simulink model "CubeX_Fast_MPC_2D"  (R2016b)
settings: Solver=FixedStepDiscrete  StartTime=0.0  StopTime=inf  FixedStep=Ts.base  RelTol=1e-3
PreLoadFcn:
  | waijung.modelPreload; % Required for working with Waijung Blockset. Do not remove.
InitFcn:
  | cubeparameters
undefined symbols (not defined in the file or in its folder): CPHA_1Edge, CPOL_Low, deg_, Duplex, FirstBit_MSB, Full, g, imu, Link, LQFP100, ST, STM32F407VG, STM32F4DISCOVERY, Ts
libraries: simulink x47, stm32f4_i2c_lib x12, stm32f4_io_lib x5, stm32f4_spi_lib x4, cube_lib x3, BC_USB x2, stm32f4_adc_lib x1, stm32f4_device_config_lib x1
(part 2 of 3)

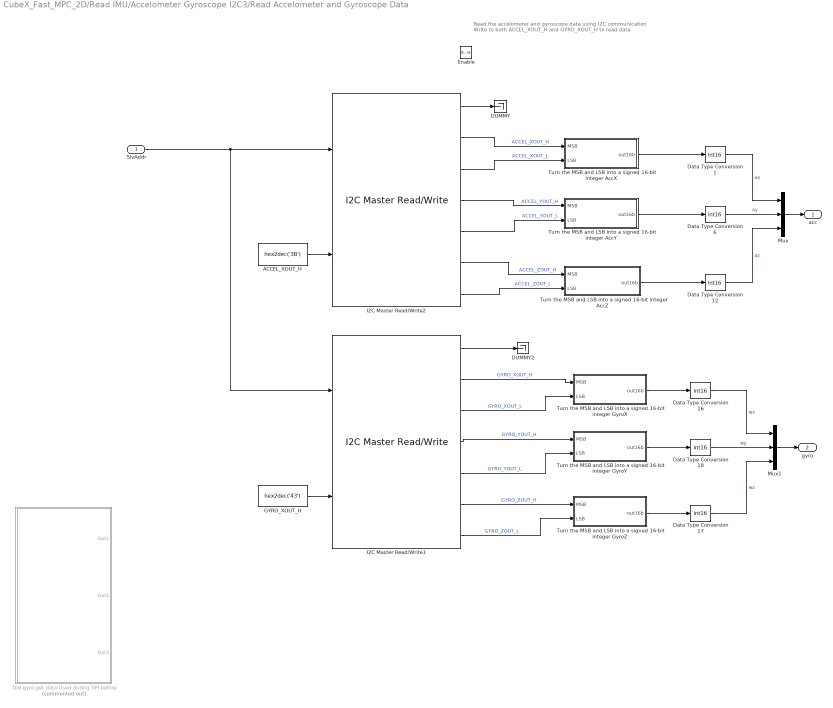
== system CubeX_Fast_MPC_2D/Read IMU/Accelometer Gyroscope I2C3/Read Accelometer and Gyroscope Data ==
  note: Read the accelometer and gyroscope data using I2C communication
      | Write to both ACCEL_XOUT_H and GYRO_XOUT_H to read data
  SlvAddr : Inport
  Enable : EnablePort
  ACCEL_XOUT_H : Constant  Value=hex2dec('3B')  OutDataTypeStr=uint8  SampleTime=-1
  DUMMY : Terminator
  DUMMY2 : Terminator
  Data Type Conversion{1,6,12,16..18} (6 alike) : DataTypeConversion  OutDataTypeStr=int16
  GYRO_XOUT_H : Constant  Value=hex2dec('43')  OutDataTypeStr=uint8  SampleTime=-1
  I2C Master Read/Write1 : stm32f4_i2c_lib/I2C Master Read//Write  configuration=Transaction  module=3  lastmodule=3  transfer=Blocking  dutycycle=TLow/THigh = 2  clkspeed=400  timeout=25  writecount=1  readcount=6  sdapin=C9  sclpin=A8  waitwritetime=0  forcestop=off  inputtypearray=[2 3 3]  outputtypearray=[7 3 3 3 3 3 3 3]  confstr="[\"C\",\"9\",\"A\",\"8\",\"1\",\"3\",\"4\",\"2\",\"I2C_DutyCycle_2\",\"0\",\"off\"]"  sampletime=Ts.IMU  sampletimestr=0.008  blockid=ReadIMUAccelometerGyroscopeI2C3ReadAccelometerandGyroscopeDataI2CMasterReadWrite1
  I2C Master Read/Write2 : stm32f4_i2c_lib/I2C Master Read//Write  configuration=Transaction  module=3  lastmodule=3  transfer=Blocking  dutycycle=TLow/THigh = 2  clkspeed=400  timeout=25  writecount=1  readcount=6  sdapin=C9  sclpin=A8  waitwritetime=0  forcestop=off  inputtypearray=[2 3 3]  outputtypearray=[7 3 3 3 3 3 3 3]  confstr="[\"C\",\"9\",\"A\",\"8\",\"1\",\"3\",\"4\",\"2\",\"I2C_DutyCycle_2\",\"0\",\"off\"]"  sampletime=Ts.IMU  sampletimestr=0.008  blockid=ReadIMUAccelometerGyroscopeI2C3ReadAccelometerandGyroscopeDataI2CMasterReadWrite2
  Mux : Mux  Inputs=3
  Mux1 : Mux  Inputs=3
  Old gyro get data Used during SPI before : Subsystem  Commented=on
  Turn the MSB and LSB into a signed 16-bit integer AccX : Subsystem
  Turn the MSB and LSB into a signed 16-bit integer AccY : Subsystem
  Turn the MSB and LSB into a signed 16-bit integer AccZ : Subsystem
  Turn the MSB and LSB into a signed 16-bit integer GyroX : Subsystem
  Turn the MSB and LSB into a signed 16-bit integer GyroY : Subsystem
  Turn the MSB and LSB into a signed 16-bit integer GyroZ : Subsystem
  acc : Outport
  gyro : Outport  Port=2
  wires:
  I2C Master Read/Write2/1 -> DUMMY/1
  Mux/1 -> acc/1
  Turn the MSB and LSB into a signed 16-bit integer AccX/1(out16b) -> Data Type Conversion1/1
  Turn the MSB and LSB into a signed 16-bit integer AccY/1(out16b) -> Data Type Conversion6/1
  Turn the MSB and LSB into a signed 16-bit integer AccZ/1(out16b) -> Data Type Conversion12/1
  Data Type Conversion1/1 -> Mux/1  "ax"
  Data Type Conversion6/1 -> Mux/2  "ay"
  Data Type Conversion12/1 -> Mux/3  "az"
  I2C Master Read/Write1/1 -> DUMMY2/1
  Mux1/1 -> gyro/1
  Turn the MSB and LSB into a signed 16-bit integer GyroX/1(out16b) -> Data Type Conversion16/1
  Turn the MSB and LSB into a signed 16-bit integer GyroY/1(out16b) -> Data Type Conversion18/1
  Turn the MSB and LSB into a signed 16-bit integer GyroZ/1(out16b) -> Data Type Conversion17/1
  Data Type Conversion16/1 -> Mux1/1  "wx"
  Data Type Conversion18/1 -> Mux1/2  "wy"
  Data Type Conversion17/1 -> Mux1/3  "wz"
  GYRO_XOUT_H/1 -> I2C Master Read/Write1/2
  ACCEL_XOUT_H/1 -> I2C Master Read/Write2/2
  SlvAddr/1 -> I2C Master Read/Write1/1, I2C Master Read/Write2/1
  I2C Master Read/Write2/2 -> Turn the MSB and LSB into a signed 16-bit integer AccX/1(MSB)  "ACCEL_XOUT_H"
  I2C Master Read/Write2/3 -> Turn the MSB and LSB into a signed 16-bit integer AccX/2(LSB)  "ACCEL_XOUT_L"
  I2C Master Read/Write2/5 -> Turn the MSB and LSB into a signed 16-bit integer AccY/2(LSB)  "ACCEL_YOUT_L"
  I2C Master Read/Write2/4 -> Turn the MSB and LSB into a signed 16-bit integer AccY/1(MSB)  "ACCEL_YOUT_H"
  I2C Master Read/Write2/6 -> Turn the MSB and LSB into a signed 16-bit integer AccZ/1(MSB)  "ACCEL_ZOUT_H"
  I2C Master Read/Write2/7 -> Turn the MSB and LSB into a signed 16-bit integer AccZ/2(LSB)  "ACCEL_ZOUT_L"
  I2C Master Read/Write1/2 -> Turn the MSB and LSB into a signed 16-bit integer GyroX/1(MSB)  "GYRO_XOUT_H"
  I2C Master Read/Write1/3 -> Turn the MSB and LSB into a signed 16-bit integer GyroX/2(LSB)  "GYRO_XOUT_L"
  I2C Master Read/Write1/4 -> Turn the MSB and LSB into a signed 16-bit integer GyroY/1(MSB)  "GYRO_YOUT_H"
  I2C Master Read/Write1/5 -> Turn the MSB and LSB into a signed 16-bit integer GyroY/2(LSB)  "GYRO_YOUT_L"
  I2C Master Read/Write1/6 -> Turn the MSB and LSB into a signed 16-bit integer GyroZ/1(MSB)  "GYRO_ZOUT_H"
  I2C Master Read/Write1/7 -> Turn the MSB and LSB into a signed 16-bit integer GyroZ/2(LSB)  "GYRO_ZOUT_L"

== system CubeX_Fast_MPC_2D/Read IMU/Magnetometer I2C1/AK8963 Init  ==
  note: See if the magnetometer is on, if not
      | set the mode to  Continuous measurement mode 2 and the output to 16 bits
      | in Write Configuration
  SlvAddr : Inport
  AK8963_CNTL : Constant  Value=hex2dec('0A')  OutDataTypeStr=uint8  SampleTime=-1
  Bitwise Operator : simulink/Logic and Bit Operations/Bitwise Operator  logicop=AND  UseBitMask=on  BitMask=bin2dec('00010110')  BitMaskRealWorld=Stored Integer
  Compare To Zero : simulink/Logic and Bit Operations/Compare To Zero  relop===  OutDataTypeStr=boolean
  I2C Master Read/Write : stm32f4_i2c_lib/I2C Master Read//Write  configuration=Transaction  module=1  lastmodule=3  transfer=Blocking  dutycycle=TLow/THigh = 2  clkspeed=400  timeout=25  writecount=1  readcount=1  sdapin=C9  sclpin=A8  waitwritetime=0  forcestop=off  inputtypearray=[2 3 3]  outputtypearray=[2 3 3]  confstr="[\"C\",\"9\",\"A\",\"8\",\"1\",\"1\",\"6\",\"0\",\"I2C_DutyCycle_2\",\"0\",\"off\"]"  sampletime=-1  sampletimestr=0.002  blockid=ReadIMUMagnetometerI2CAK8963InitI2CMasterReadWrite
  Logical Operator : Logic  AllPortsSameDT=off  OutDataTypeStr=boolean
  Logical Operator1 : Logic  AllPortsSameDT=off  OutDataTypeStr=boolean
  Logical Operator2 : Logic  Operator=NOT  AllPortsSameDT=off  OutDataTypeStr=boolean
  Write Configuration : Subsystem
  READY : Outport
  wires:
  SlvAddr/1 -> Write Configuration/1(SlvAddr), I2C Master Read/Write/1
  AK8963_CNTL/1 -> Write Configuration/2(RegAddr), I2C Master Read/Write/2
  I2C Master Read/Write/1 -> Compare To Zero/1
  Logical Operator/1 -> READY/1
  Bitwise Operator/1 -> Logical Operator2/1, Logical Operator/2
  Compare To Zero/1 -> Logical Operator/1, Logical Operator1/1
  I2C Master Read/Write/2 -> Bitwise Operator/1
  Logical Operator2/1 -> Logical Operator1/2
  Logical Operator1/1 -> Write Configuration/Enable

== system CubeX_Fast_MPC_2D/Read IMU/Magnetometer I2C1/Magnetometer Data Ready  ==
  note: Check if magnetometer data is ready
  SlvAddr : Inport
  Enable : EnablePort
  AK8963_ST1 : Constant  Value=hex2dec('02')  OutDataTypeStr=uint8  SampleTime=-1
  Bitwise Operator : simulink/Logic and Bit Operations/Bitwise Operator  logicop=AND  UseBitMask=on  BitMask=bin2dec('00000001')  BitMaskRealWorld=Stored Integer
  Compare To Zero : simulink/Logic and Bit Operations/Compare To Zero  relop===  OutDataTypeStr=boolean
  I2C Master Read/Write : stm32f4_i2c_lib/I2C Master Read//Write  configuration=Transaction  module=1  lastmodule=3  transfer=Blocking  dutycycle=TLow/THigh = 2  clkspeed=400  timeout=25  writecount=1  readcount=1  sdapin=C9  sclpin=A8  waitwritetime=0  forcestop=off  inputtypearray=[2 3 3]  outputtypearray=[2 3 3]  confstr="[\"C\",\"9\",\"A\",\"8\",\"1\",\"1\",\"6\",\"0\",\"I2C_DutyCycle_2\",\"0\",\"off\"]"  sampletime=-1  sampletimestr=0.002  blockid=ReadIMUMagnetometerI2CMagnetometerDataReadyI2CMasterReadWrite
  Logical Operator : Logic  AllPortsSameDT=off  OutDataTypeStr=boolean
  READY : Outport
  wires:
  SlvAddr/1 -> I2C Master Read/Write/1
  AK8963_ST1/1 -> I2C Master Read/Write/2
  I2C Master Read/Write/2 -> Bitwise Operator/1
  I2C Master Read/Write/1 -> Compare To Zero/1
  Compare To Zero/1 -> Logical Operator/1
  Bitwise Operator/1 -> Logical Operator/2
  Logical Operator/1 -> READY/1

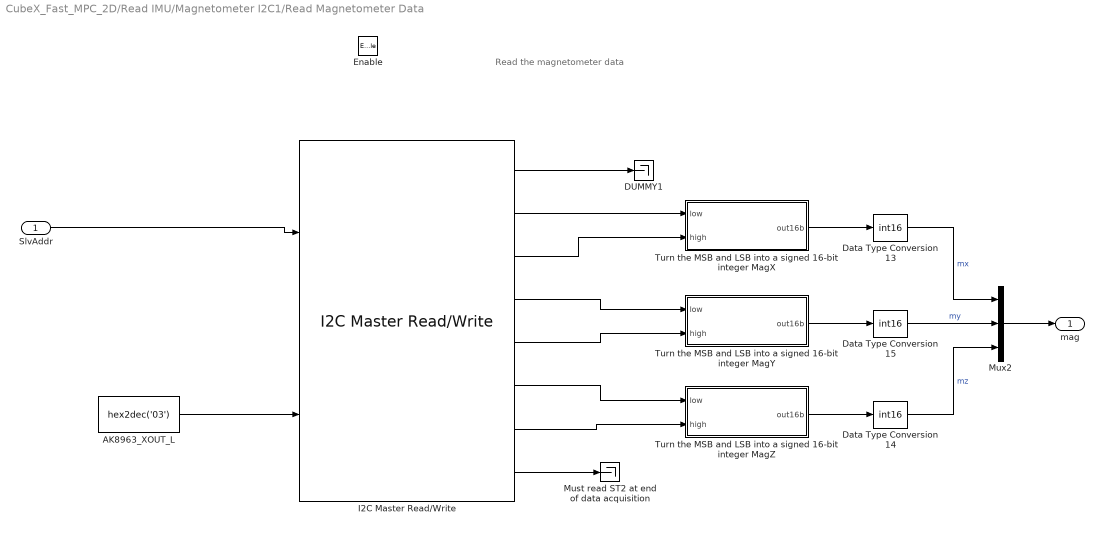
== system CubeX_Fast_MPC_2D/Read IMU/Magnetometer I2C1/Read Magnetometer Data ==
  note: Read the magnetometer data
  "SlvAddr " : Inport
  Enable : EnablePort
  AK8963_XOUT_L : Constant  Value=hex2dec('03')  OutDataTypeStr=uint8  SampleTime=-1
  DUMMY1 : Terminator
  Data Type Conversion13 : DataTypeConversion  OutDataTypeStr=int16
  Data Type Conversion14 : DataTypeConversion  OutDataTypeStr=int16
  Data Type Conversion15 : DataTypeConversion  OutDataTypeStr=int16
  I2C Master Read/Write : stm32f4_i2c_lib/I2C Master Read//Write  configuration=Transaction  module=1  lastmodule=3  transfer=Blocking  dutycycle=TLow/THigh = 2  clkspeed=400  timeout=25  writecount=1  readcount=7  sdapin=C9  sclpin=A8  waitwritetime=0  forcestop=off  inputtypearray=[2 3 3]  outputtypearray=[8 3 3 3 3 3 3 3 3]  confstr="[\"C\",\"9\",\"A\",\"8\",\"1\",\"1\",\"6\",\"0\",\"I2C_DutyCycle_2\",\"0\",\"off\"]"  sampletime=-1  sampletimestr=0.002  blockid=ReadIMUMagnetometerI2CReadMagnetometerDataI2CMasterReadWrite
  "Must read ST2 at end of data acquisition  " : Terminator
  Mux2 : Mux  Inputs=3
  Turn the MSB and LSB into a signed 16-bit integer MagX : Subsystem
  Turn the MSB and LSB into a signed 16-bit integer MagY : Subsystem
  Turn the MSB and LSB into a signed 16-bit integer MagZ : Subsystem
  mag : Outport
  wires:
  Turn the MSB and LSB into a signed 16-bit integer MagX/1(out16b) -> Data Type Conversion13/1
  Turn the MSB and LSB into a signed 16-bit integer MagY/1(out16b) -> Data Type Conversion15/1
  Turn the MSB and LSB into a signed 16-bit integer MagZ/1(out16b) -> Data Type Conversion14/1
  Data Type Conversion13/1 -> Mux2/1  "mx"
  Data Type Conversion15/1 -> Mux2/2  "my"
  Data Type Conversion14/1 -> Mux2/3  "mz"
  AK8963_XOUT_L/1 -> I2C Master Read/Write/2
  I2C Master Read/Write/1 -> DUMMY1/1
  "SlvAddr "/1 -> I2C Master Read/Write/1
  Mux2/1 -> mag/1
  I2C Master Read/Write/8 -> "Must read ST2 at end of data acquisition  "/1
  I2C Master Read/Write/3 -> Turn the MSB and LSB into a signed 16-bit integer MagX/2(high)
  I2C Master Read/Write/2 -> Turn the MSB and LSB into a signed 16-bit integer MagX/1(low)
  I2C Master Read/Write/4 -> Turn the MSB and LSB into a signed 16-bit integer MagY/1(low)
  I2C Master Read/Write/5 -> Turn the MSB and LSB into a signed 16-bit integer MagY/2(high)
  I2C Master Read/Write/6 -> Turn the MSB and LSB into a signed 16-bit integer MagZ/1(low)
  I2C Master Read/Write/7 -> Turn the MSB and LSB into a signed 16-bit integer MagZ/2(high)

== system CubeX_Fast_MPC_2D/Read IMU/SPI3/Turn the MSB and LSB into a signed 16-bit integer AccX ==
  MSB : Inport
  LSB : Inport  Port=2
  Bitwise Operator2 : simulink/Logic and Bit Operations/Bitwise Operator  logicop=OR  UseBitMask=off  NumInputPorts=2  BitMask=bin2dec('11011001')  BitMaskRealWorld=Stored Integer
  Data Type Conversion6 : DataTypeConversion  OutDataTypeStr=uint16
  Data Type Conversion7 : DataTypeConversion  OutDataTypeStr=uint16
  Shift Arithmetic2 : ArithShift  BitShiftNumber=-8
  out16b : Outport
  wires:
  LSB/1 -> Data Type Conversion6/1
  Bitwise Operator2/1 -> out16b/1
  MSB/1 -> Data Type Conversion7/1
  Data Type Conversion7/1 -> Shift Arithmetic2/1
  Data Type Conversion6/1 -> Bitwise Operator2/2
  Shift Arithmetic2/1 -> Bitwise Operator2/1

== system CubeX_Fast_MPC_2D/Read IMU/SPI3/Turn the MSB and LSB into a signed 16-bit integer AccY ==
  MSB : Inport
  LSB : Inport  Port=2
  Bitwise Operator2 : simulink/Logic and Bit Operations/Bitwise Operator  logicop=OR  UseBitMask=off  NumInputPorts=2  BitMask=bin2dec('11011001')  BitMaskRealWorld=Stored Integer
  Data Type Conversion6 : DataTypeConversion  OutDataTypeStr=int16
  Data Type Conversion7 : DataTypeConversion  OutDataTypeStr=int16
  Shift Arithmetic2 : ArithShift  BitShiftNumber=-8
  out16b : Outport
  wires:
  LSB/1 -> Data Type Conversion6/1
  Bitwise Operator2/1 -> out16b/1
  MSB/1 -> Data Type Conversion7/1
  Data Type Conversion7/1 -> Shift Arithmetic2/1
  Data Type Conversion6/1 -> Bitwise Operator2/2
  Shift Arithmetic2/1 -> Bitwise Operator2/1

== system CubeX_Fast_MPC_2D/Read IMU/SPI3/Turn the MSB and LSB into a signed 16-bit integer AccZ ==
  MSB : Inport
  LSB : Inport  Port=2
  Bitwise Operator2 : simulink/Logic and Bit Operations/Bitwise Operator  logicop=OR  UseBitMask=off  NumInputPorts=2  BitMask=bin2dec('11011001')  BitMaskRealWorld=Stored Integer
  Data Type Conversion6 : DataTypeConversion  OutDataTypeStr=int16
  Data Type Conversion7 : DataTypeConversion  OutDataTypeStr=int16
  Shift Arithmetic2 : ArithShift  BitShiftNumber=-8
  out16b : Outport
  wires:
  LSB/1 -> Data Type Conversion6/1
  Bitwise Operator2/1 -> out16b/1
  MSB/1 -> Data Type Conversion7/1
  Data Type Conversion7/1 -> Shift Arithmetic2/1
  Data Type Conversion6/1 -> Bitwise Operator2/2
  Shift Arithmetic2/1 -> Bitwise Operator2/1

== system CubeX_Fast_MPC_2D/Read IMU/SPI3/Turn the MSB and LSB into a signed 16-bit integer GyroX ==
  MSB : Inport
  LSB : Inport  Port=2
  Bitwise Operator2 : simulink/Logic and Bit Operations/Bitwise Operator  logicop=OR  UseBitMask=off  NumInputPorts=2  BitMask=bin2dec('11011001')  BitMaskRealWorld=Stored Integer
  Data Type Conversion1 : DataTypeConversion  OutDataTypeStr=int16
  Data Type Conversion7 : DataTypeConversion  OutDataTypeStr=int16
  Shift Arithmetic2 : ArithShift  BitShiftNumber=-8
  out16b : Outport
  wires:
  MSB/1 -> Data Type Conversion7/1
  Data Type Conversion7/1 -> Shift Arithmetic2/1
  Shift Arithmetic2/1 -> Bitwise Operator2/1
  LSB/1 -> Data Type Conversion1/1
  Data Type Conversion1/1 -> Bitwise Operator2/2
  Bitwise Operator2/1 -> out16b/1

== system CubeX_Fast_MPC_2D/Read IMU/SPI3/Turn the MSB and LSB into a signed 16-bit integer GyroY ==
  MSB : Inport
  LSB : Inport  Port=2
  Bitwise Operator2 : simulink/Logic and Bit Operations/Bitwise Operator  logicop=OR  UseBitMask=off  NumInputPorts=2  BitMask=bin2dec('11011001')  BitMaskRealWorld=Stored Integer
  Data Type Conversion6 : DataTypeConversion  OutDataTypeStr=uint16
  Data Type Conversion7 : DataTypeConversion  OutDataTypeStr=uint16
  Shift Arithmetic2 : ArithShift  BitShiftNumber=-8
  out16b : Outport
  wires:
  LSB/1 -> Data Type Conversion6/1
  Bitwise Operator2/1 -> out16b/1
  MSB/1 -> Data Type Conversion7/1
  Data Type Conversion7/1 -> Shift Arithmetic2/1
  Data Type Conversion6/1 -> Bitwise Operator2/2
  Shift Arithmetic2/1 -> Bitwise Operator2/1

== system CubeX_Fast_MPC_2D/Read IMU/SPI3/Turn the MSB and LSB into a signed 16-bit integer GyroZ ==
  MSB : Inport
  LSB : Inport  Port=2
  Bitwise Operator2 : simulink/Logic and Bit Operations/Bitwise Operator  logicop=OR  UseBitMask=off  NumInputPorts=2  BitMask=bin2dec('11011001')  BitMaskRealWorld=Stored Integer
  Data Type Conversion6 : DataTypeConversion  OutDataTypeStr=uint16
  Data Type Conversion7 : DataTypeConversion  OutDataTypeStr=uint16
  Shift Arithmetic2 : ArithShift  BitShiftNumber=-8
  out16b : Outport
  wires:
  LSB/1 -> Data Type Conversion6/1
  Bitwise Operator2/1 -> out16b/1
  MSB/1 -> Data Type Conversion7/1
  Data Type Conversion7/1 -> Shift Arithmetic2/1
  Data Type Conversion6/1 -> Bitwise Operator2/2
  Shift Arithmetic2/1 -> Bitwise Operator2/1

== system CubeX_Fast_MPC_2D/Read IMU/Subsystem/Subsystem ==
  Enable : EnablePort
  SPI Master Read/Write1 : stm32f4_spi_lib/SPI Master Read//Write  configuration=Transaction  module=3  mode=Read/ Write  lastmodule=1  direction=Full-Duplex  dataformat=8bit/ FirstBit_MSB  prescaler=4  cpolcpha=CPOL_Low/ CPHA_1Edge  datacount=2  nssmode=Custom  nsspin=Not used  softnssport=E  softnsspin=0  sckpin=A5  misopin=A6  mosipin=A7  inputtypearray=[2 3 3]  outputtypearray=[3 7 3 3]  confstr="[\"SPI_Direction_2Lines_FullDuplex\",\"8b\",\"MSB\",\"Low\",\"1Edge\",\"4\",\"Soft\",\"0\",\"x\",\"x\",\"0\",\"x\",\"x\",\"1\",\"A\",\"5\",\"1\",\"A\",\"6\",\"1\",\"A\",\"7\",\"1\",\"0\",\"0\",\"0\",\"0\",\"0\",\"0\",\"0\",\"0\",\"PP\",\"0\",\"UP\"]"  sampletime=0.002  sampletimestr=0.002  blockid=ReadIMUSubsystemSubsystemSPIMasterReadWrite1
  Terminator : Terminator
  Terminator1 : Terminator
  Terminator2 : Terminator
  USER_CTRL : Constant  Value=hex2dec('6A')  OutDataTypeStr=uint8  SampleTime=-1
  USER_CTRL1 : Constant  Value=hex2dec('10')  OutDataTypeStr=uint8  SampleTime=-1
  wires:
  SPI Master Read/Write1/3 -> Terminator/1
  SPI Master Read/Write1/2 -> Terminator1/1
  SPI Master Read/Write1/1 -> Terminator2/1
  USER_CTRL/1 -> SPI Master Read/Write1/1
  USER_CTRL1/1 -> SPI Master Read/Write1/2

== system CubeX_Fast_MPC_2D/Read IMU/Accelometer Gyroscope I2C1/MPU9250 Init/Write Configuration ==
  note: Enable BYPSS_EN in INT_PIN_CFG register to be able to read magnetometer trough I2C
  SlvAddr : Inport
  Enable : EnablePort
  BYPASS_EN : Constant  Value=hex2dec('02')  OutDataTypeStr=uint8  SampleTime=-1
  I2C Master Read/Write1 : stm32f4_i2c_lib/I2C Master Read//Write  configuration=Transaction  module=1  lastmodule=3  transfer=Blocking  dutycycle=TLow/THigh = 2  clkspeed=400  timeout=25  writecount=2  readcount=0  sdapin=C9  sclpin=A8  waitwritetime=0  forcestop=off  inputtypearray=[3 3 3 3]  outputtypearray=[1 3]  confstr="[\"C\",\"9\",\"A\",\"8\",\"1\",\"1\",\"6\",\"0\",\"I2C_DutyCycle_2\",\"0\",\"off\"]"  sampletime=-1  sampletimestr=0.008  blockid=ReadIMUAccelometerGyroscopeI2C1MPU9250InitWriteConfigurationI2CMasterReadWrite1
  INT_PIN_CFG1 : Constant  Value=hex2dec('37')  OutDataTypeStr=uint8  SampleTime=-1
  Terminator : Terminator
  wires:
  I2C Master Read/Write1/1 -> Terminator/1
  BYPASS_EN/1 -> I2C Master Read/Write1/3
  INT_PIN_CFG1/1 -> I2C Master Read/Write1/2
  SlvAddr/1 -> I2C Master Read/Write1/1

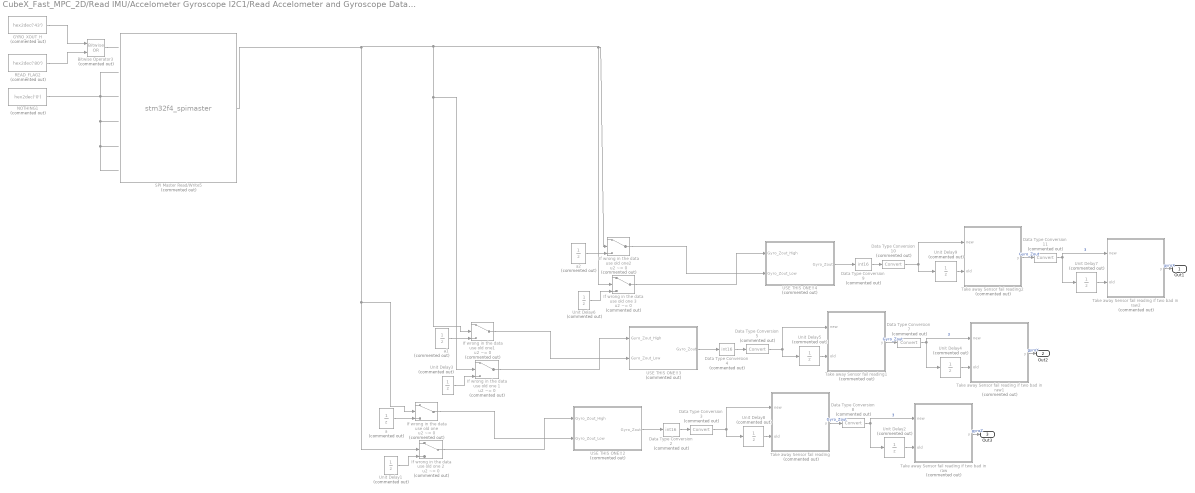
== system CubeX_Fast_MPC_2D/Read IMU/Accelometer Gyroscope I2C1/Read Accelometer and Gyroscope Data/Old gyro get data Used during SPI before ==
  " a" : UnitDelay  Commented=on  SampleTime=-1
  " a1" : UnitDelay  Commented=on  SampleTime=-1
  " a2" : UnitDelay  Commented=on  SampleTime=-1
  Bitwise Operator3 : simulink/Logic and Bit Operations/Bitwise Operator  Commented=on  logicop=OR  UseBitMask=off  NumInputPorts=2  BitMask=bin2dec('11011001')  BitMaskRealWorld=Stored Integer
  Data Type Conversion{3,5,7..8,10..11} (6 alike) : DataTypeConversion  Commented=on
  Data Type Conversion2 : DataTypeConversion  Commented=on  OutDataTypeStr=int16
  Data Type Conversion4 : DataTypeConversion  Commented=on  OutDataTypeStr=int16
  Data Type Conversion9 : DataTypeConversion  Commented=on  OutDataTypeStr=int16
  GYRO_XOUT_H : Constant  Commented=on  Value=hex2dec('43')  OutDataTypeStr=uint8
  If wrong in the data use old one : Switch  Commented=on  Criteria=u2 ~= 0
  If wrong in the data use old one 1 : Switch  Commented=on  Criteria=u2 ~= 0
  If wrong in the data use old one 2 : Switch  Commented=on  Criteria=u2 ~= 0
  If wrong in the data use old one 3 : Switch  Commented=on  Criteria=u2 ~= 0
  If wrong in the data use old one1 : Switch  Commented=on  Criteria=u2 ~= 0
  If wrong in the data use old one2 : Switch  Commented=on  Criteria=u2 ~= 0
  NOTHING1 : Constant  Commented=on  Value=hex2dec('0')  OutDataTypeStr=uint8
  READ_FLAG2 : Constant  Commented=on  Value=hex2dec('80')  OutDataTypeStr=uint8
  SPI Master Read/Write5 : S-Function  Commented=on  FunctionName=stm32f4_spimaster  Parameters=mode,configuration,module,datacount,inputtypearray,outputtypearray,confstr,sampletime,sampletimestr,blockid  SFunctionDeploymentMode=off  EnableBusSupport=off  mask(stm32f4_spimaster){configuration=Transaction, module=3, mode=Read/ Write, lastmodule=1, direction=Full-Duplex, dataformat=8bit/ FirstBit_MSB, prescaler=4, cpolcpha=CPOL_Low/ CPHA_1Edge, datacount='Could not find SPI Master Setup block for module 3', nssmode=Custom, nsspin=Not used, softnssport=E, softnsspin=0, sckpin=A5, misopin=A6, mosipin=A7, inputtypearray=[0], outputtypearray=[1 7], confstr=["SPI_Direction_2Lines_FullDuplex","8b","MSB","Low","1Edge","4","Soft","0","x","x","0","x","x","1","A","5","1","A","6","1","A","7","1","0","0","0","0","0","0","0","0","PP","0","UP"], sampletime=-1, sampletimestr=-1, blockid=AccelometerGyroscopeI2CReadAccelometerandGyroscopeDataOldgyrogetdataUsedduringSPIbeforeSPIMasterReadWrite5}
      mask prompts: module "SPI Module:"; lastmodule "Last module:"; dataformat "Data format:"; prescaler "Buad rate prescaler: Pclk/"; cpolcpha "Clock polarity (CPOL)/ Clock phase (CPHA):"; datacount "Data Read/Write count:"; nssmode "Slave/chip select (nSS, nCS) mode"; nsspin "Slave/chip select (nSS, nCS) pin"; softnssport "Slave/chip select port (nSS, nCS)"; softnsspin "Slave/chip select pin (nSS, nCS)"; sckpin "SCLK pin:"; misopin "MISO pin:"; mosipin "MOSI pin:"; inputtypearray "Input type array"; outputtypearray "Output type array"; confstr "Configuration string"; sampletime "Sample time (sec)"; sampletimestr "Compiled sample time (sec) in string"
      mask help:
      | Status:
      |  0 - Success.
      |  Otherwise - Fail.
      mask init:
      | stm32f4_spimaster_callback('init');
      mask Help: web(fullfile(waijungdocroot,'stm32f4_spimaster_readwrite.htm'), '-browser')
      mask TypeOptions configuration: Setup | Transaction
      mask Callback configuration: stm32f4_spimaster_callback('configuration');
      mask TypeOptions module: 1 | 2 | 3
      mask Callback module: stm32f4_spimaster_callback('module');
      mask TypeOptions mode: Read/ Write | Read | Write
      mask Callback mode: stm32f4_spimaster_callback('mode');
      mask TypeOptions direction: Full-Duplex | Half-Duplex_Tx | Half-Duplex_Rx
      mask Callback direction: stm32f4_spimaster_callback('direction');
      mask TypeOptions dataformat: 8bit/ FirstBit_MSB | 8bit/ FirstBit_LSB | 16bit/ FirstBit_MSB | 16bit/ FirstBit_LSB
      mask TypeOptions prescaler: 2 | 4 | 8 | 16 | 32 | 64 | 128 | 256
      mask TypeOptions cpolcpha: CPOL_Low/ CPHA_1Edge | CPOL_Low/ CPHA_2Edge | CPOL_High/ CPHA_1Edge | CPOL_High/ CPHA_2Edge
      mask Callback datacount: stm32f4_spimaster_callback('datacount');
      mask TypeOptions nssmode: Hardware | Software | Custom
      mask Callback nssmode: stm32f4_spimaster_callback('nssmode');
      mask TypeOptions nsspin: Not used | A4 | A15
      mask TypeOptions softnssport: A | B | C | D | E | F | G | H | I
      mask TypeOptions softnsspin: 0 | 1 | 2 | 3 | 4 | 5 | 6 | 7 | 8 | 9 | 10 | 11 | 12 | 13 | 14 | 15
      mask TypeOptions sckpin: Not used | A5 | B3
      mask TypeOptions misopin: Not used | A6 | B4
      mask TypeOptions mosipin: Not used | A7 | B5
      mask Callback confstr: stm32f4_spimaster_callback('confstr');
      mask Callback sampletime: stm32f4_spimaster_callback('sampletime');
      mask Callback sampletimestr: stm32f4_spimaster_callback('sampletimestr');
      mask Callback blockid: stm32f4_spimaster_callback('blockid');
      mask Display: text(0.5, 0.5, 'Module: SPI3 (Master)\nRead/ Write\nTs (sec): -1','ver','middle','hor','center');port_label('output', 1,'Status');
  Take away Sensor fail reading : MATLAB Function  Commented=on  TreatAsAtomicUnit=on
  Take away Sensor fail reading if two bad in raw : MATLAB Function  Commented=on  TreatAsAtomicUnit=on
  Take away Sensor fail reading if two bad in raw1 : MATLAB Function  Commented=on  TreatAsAtomicUnit=on
  Take away Sensor fail reading if two bad in raw2 : MATLAB Function  Commented=on  TreatAsAtomicUnit=on
  Take away Sensor fail reading1 : MATLAB Function  Commented=on  TreatAsAtomicUnit=on
  Take away Sensor fail reading2 : MATLAB Function  Commented=on  TreatAsAtomicUnit=on
  USE THIS ONE!!2 : Subsystem  Commented=on
  USE THIS ONE!!3 : Subsystem  Commented=on
  USE THIS ONE!!4 : Subsystem  Commented=on
  Unit Delay1 : UnitDelay  Commented=on  SampleTime=-1
  Unit Delay{2,4..5,7..9} (6 alike) : UnitDelay  Commented=on  InitialCondition=-40.45  SampleTime=-1
  Unit Delay3 : UnitDelay  Commented=on  SampleTime=-1
  Unit Delay6 : UnitDelay  Commented=on  SampleTime=-1
  Out1 : Outport
  Out2 : Outport  Port=2
  Out3 : Outport  Port=3
  wires:
  Data Type Conversion8/1 -> Unit Delay2/1, Take away Sensor fail reading if two bad in raw/1(new)  "3"
  Bitwise Operator3/1 -> ?
  USE THIS ONE!!2/1(Gyro_Zout) -> Data Type Conversion2/1
  GYRO_XOUT_H/1 -> Bitwise Operator3/1
  Unit Delay8/1 -> Take away Sensor fail reading/2(old)
  ? -> If wrong in the data use old one 2/1, Unit Delay1/1
  READ_FLAG2/1 -> Bitwise Operator3/2
  If wrong in the data use old one 2/1 -> USE THIS ONE!!2/1("Gyro_Zout_High ")
  If wrong in the data use old one/1 -> USE THIS ONE!!2/2(Gyro_Zout_Low)
  ? -> " a"/1, If wrong in the data use old one/1  "Gyro_zou_Lowt"
  " a"/1 -> If wrong in the data use old one/3
  Data Type Conversion2/1 -> Data Type Conversion3/1
  NOTHING1/1 -> ?
  Unit Delay1/1 -> If wrong in the data use old one 2/3
  Take away Sensor fail reading/1(y) -> Data Type Conversion8/1  "Gyro_Zout"
  Unit Delay2/1 -> Take away Sensor fail reading if two bad in raw/2(old)
  Unit Delay7/1 -> Take away Sensor fail reading if two bad in raw2/2(old)
  If wrong in the data use old one1/1 -> USE THIS ONE!!3/2(Gyro_Zout_Low)
  ? -> Unit Delay3/1, If wrong in the data use old one 1/1  "Gyro_zou_Lowt"
  " a2"/1 -> If wrong in the data use old one2/3
  Take away Sensor fail reading2/1(y) -> Data Type Conversion11/1  "Gyro_Zout"
  Data Type Conversion10/1 -> Take away Sensor fail reading2/1(new), Unit Delay9/1
  Data Type Conversion11/1 -> Unit Delay7/1, Take away Sensor fail reading if two bad in raw2/1(new)  "3"
  Unit Delay5/1 -> Take away Sensor fail reading1/2(old)
  SPI Master Read/Write5/1 -> If wrong in the data use old one2/2, If wrong in the data use old one 3/2, If wrong in the data use old one 1/2, If wrong in the data use old one1/2, If wrong in the data use old one 2/2, If wrong in the data use old one/2
  ? -> " a2"/1, If wrong in the data use old one2/1  "Gyro_zou_Lowt"
  ? -> " a1"/1, If wrong in the data use old one1/1  "Gyro_zou_Lowt"
  Data Type Conversion7/1 -> Unit Delay4/1, Take away Sensor fail reading if two bad in raw1/1(new)  "3"
  Data Type Conversion3/1 -> Take away Sensor fail reading/1(new), Unit Delay8/1
  Data Type Conversion4/1 -> Data Type Conversion5/1
  Data Type Conversion9/1 -> Data Type Conversion10/1
  USE THIS ONE!!3/1(Gyro_Zout) -> Data Type Conversion4/1
  " a1"/1 -> If wrong in the data use old one1/3
  Unit Delay6/1 -> If wrong in the data use old one 3/3
  USE THIS ONE!!4/1(Gyro_Zout) -> Data Type Conversion9/1
  If wrong in the data use old one 1/1 -> USE THIS ONE!!3/1("Gyro_Zout_High ")
  If wrong in the data use old one2/1 -> USE THIS ONE!!4/2(Gyro_Zout_Low)
  Unit Delay3/1 -> If wrong in the data use old one 1/3
  Data Type Conversion5/1 -> Take away Sensor fail reading1/1(new), Unit Delay5/1
  ? -> If wrong in the data use old one 3/1, Unit Delay6/1  "Gyro_zou_Lowt"
  If wrong in the data use old one 3/1 -> USE THIS ONE!!4/1("Gyro_Zout_High ")
  Unit Delay9/1 -> Take away Sensor fail reading2/2(old)
  Unit Delay4/1 -> Take away Sensor fail reading if two bad in raw1/2(old)
  Take away Sensor fail reading1/1(y) -> Data Type Conversion7/1  "Gyro_Zout"
  Take away Sensor fail reading if two bad in raw2/1(y) -> Out1/1  "gyroX"
  Take away Sensor fail reading if two bad in raw/1(y) -> Out3/1  "gyroZ"
  Take away Sensor fail reading if two bad in raw1/1(y) -> Out2/1  "gyroY"

== system CubeX_Fast_MPC_2D/Read IMU/Accelometer Gyroscope I2C1/Read Accelometer and Gyroscope Data/Turn the MSB and LSB into a signed 16-bit integer AccX ==
  note: Bitshift up the MSB bits and bitwise OR the LSB
      | into a int16
  MSB : Inport
  LSB : Inport  Port=2
  Bitwise Operator2 : simulink/Logic and Bit Operations/Bitwise Operator  logicop=OR  UseBitMask=off  NumInputPorts=2  BitMask=bin2dec('11011001')  BitMaskRealWorld=Stored Integer
  Data Type Conversion6 : DataTypeConversion  OutDataTypeStr=uint16
  Data Type Conversion7 : DataTypeConversion  OutDataTypeStr=uint16
  Shift Arithmetic2 : ArithShift  BitShiftNumber=-8
  out16b : Outport
  wires:
  LSB/1 -> Data Type Conversion6/1
  Bitwise Operator2/1 -> out16b/1
  MSB/1 -> Data Type Conversion7/1
  Data Type Conversion7/1 -> Shift Arithmetic2/1
  Data Type Conversion6/1 -> Bitwise Operator2/2
  Shift Arithmetic2/1 -> Bitwise Operator2/1

== system CubeX_Fast_MPC_2D/Read IMU/Accelometer Gyroscope I2C1/Read Accelometer and Gyroscope Data/Turn the MSB and LSB into a signed 16-bit integer AccY ==
  note: Bitshift up the MSB bits and bitwise OR the LSB
      | into a int16
  MSB : Inport
  LSB : Inport  Port=2
  Bitwise Operator2 : simulink/Logic and Bit Operations/Bitwise Operator  logicop=OR  UseBitMask=off  NumInputPorts=2  BitMask=bin2dec('11011001')  BitMaskRealWorld=Stored Integer
  Data Type Conversion6 : DataTypeConversion  OutDataTypeStr=uint16
  Data Type Conversion7 : DataTypeConversion  OutDataTypeStr=uint16
  Shift Arithmetic2 : ArithShift  BitShiftNumber=-8
  out16b : Outport
  wires:
  LSB/1 -> Data Type Conversion6/1
  Bitwise Operator2/1 -> out16b/1
  MSB/1 -> Data Type Conversion7/1
  Data Type Conversion7/1 -> Shift Arithmetic2/1
  Data Type Conversion6/1 -> Bitwise Operator2/2
  Shift Arithmetic2/1 -> Bitwise Operator2/1

== system CubeX_Fast_MPC_2D/Read IMU/Accelometer Gyroscope I2C1/Read Accelometer and Gyroscope Data/Turn the MSB and LSB into a signed 16-bit integer AccZ ==
  note: Bitshift up the MSB bits and bitwise OR the LSB
      | into a int16
  MSB : Inport
  LSB : Inport  Port=2
  Bitwise Operator2 : simulink/Logic and Bit Operations/Bitwise Operator  logicop=OR  UseBitMask=off  NumInputPorts=2  BitMask=bin2dec('11011001')  BitMaskRealWorld=Stored Integer
  Data Type Conversion6 : DataTypeConversion  OutDataTypeStr=uint16
  Data Type Conversion7 : DataTypeConversion  OutDataTypeStr=uint16
  Shift Arithmetic2 : ArithShift  BitShiftNumber=-8
  out16b : Outport
  wires:
  LSB/1 -> Data Type Conversion6/1
  Bitwise Operator2/1 -> out16b/1
  MSB/1 -> Data Type Conversion7/1
  Data Type Conversion7/1 -> Shift Arithmetic2/1
  Data Type Conversion6/1 -> Bitwise Operator2/2
  Shift Arithmetic2/1 -> Bitwise Operator2/1

== system CubeX_Fast_MPC_2D/Read IMU/Accelometer Gyroscope I2C1/Read Accelometer and Gyroscope Data/Turn the MSB and LSB into a signed 16-bit integer GyroX ==
  note: Bitshift up the MSB bits and bitwise OR the LSB
      | into a int16
  MSB : Inport
  LSB : Inport  Port=2
  Bitwise Operator2 : simulink/Logic and Bit Operations/Bitwise Operator  logicop=OR  UseBitMask=off  NumInputPorts=2  BitMask=bin2dec('11011001')  BitMaskRealWorld=Stored Integer
  Data Type Conversion6 : DataTypeConversion  OutDataTypeStr=uint16
  Data Type Conversion7 : DataTypeConversion  OutDataTypeStr=uint16
  Shift Arithmetic2 : ArithShift  BitShiftNumber=-8
  out16b : Outport
  wires:
  LSB/1 -> Data Type Conversion6/1
  Bitwise Operator2/1 -> out16b/1
  MSB/1 -> Data Type Conversion7/1
  Data Type Conversion7/1 -> Shift Arithmetic2/1
  Data Type Conversion6/1 -> Bitwise Operator2/2
  Shift Arithmetic2/1 -> Bitwise Operator2/1

== system CubeX_Fast_MPC_2D/Read IMU/Accelometer Gyroscope I2C1/Read Accelometer and Gyroscope Data/Turn the MSB and LSB into a signed 16-bit integer GyroY ==
  note: Bitshift up the MSB bits and bitwise OR the LSB
      | into a int16
  MSB : Inport
  LSB : Inport  Port=2
  Bitwise Operator2 : simulink/Logic and Bit Operations/Bitwise Operator  logicop=OR  UseBitMask=off  NumInputPorts=2  BitMask=bin2dec('11011001')  BitMaskRealWorld=Stored Integer
  Data Type Conversion6 : DataTypeConversion  OutDataTypeStr=uint16
  Data Type Conversion7 : DataTypeConversion  OutDataTypeStr=uint16
  Shift Arithmetic2 : ArithShift  BitShiftNumber=-8
  out16b : Outport
  wires:
  LSB/1 -> Data Type Conversion6/1
  Bitwise Operator2/1 -> out16b/1
  MSB/1 -> Data Type Conversion7/1
  Data Type Conversion7/1 -> Shift Arithmetic2/1
  Data Type Conversion6/1 -> Bitwise Operator2/2
  Shift Arithmetic2/1 -> Bitwise Operator2/1

== system CubeX_Fast_MPC_2D/Read IMU/Accelometer Gyroscope I2C1/Read Accelometer and Gyroscope Data/Turn the MSB and LSB into a signed 16-bit integer GyroZ ==
  note: Bitshift up the MSB bits and bitwise OR the LSB
      | into a int16
  MSB : Inport
  LSB : Inport  Port=2
  Bitwise Operator2 : simulink/Logic and Bit Operations/Bitwise Operator  logicop=OR  UseBitMask=off  NumInputPorts=2  BitMask=bin2dec('11011001')  BitMaskRealWorld=Stored Integer
  Data Type Conversion6 : DataTypeConversion  OutDataTypeStr=uint16
  Data Type Conversion7 : DataTypeConversion  OutDataTypeStr=uint16
  Shift Arithmetic2 : ArithShift  BitShiftNumber=-8
  out16b : Outport
  wires:
  LSB/1 -> Data Type Conversion6/1
  Bitwise Operator2/1 -> out16b/1
  MSB/1 -> Data Type Conversion7/1
  Data Type Conversion7/1 -> Shift Arithmetic2/1
  Data Type Conversion6/1 -> Bitwise Operator2/2
  Shift Arithmetic2/1 -> Bitwise Operator2/1

== system CubeX_Fast_MPC_2D/Read IMU/Accelometer Gyroscope I2C3/MPU9250 Init/Write Configuration ==
  note: Enable BYPSS_EN in INT_PIN_CFG register to be able to read magnetometer trough I2C
  SlvAddr : Inport
  Enable : EnablePort
  BYPASS_EN : Constant  Value=hex2dec('02')  OutDataTypeStr=uint8  SampleTime=-1
  I2C Master Read/Write1 : stm32f4_i2c_lib/I2C Master Read//Write  configuration=Transaction  module=3  lastmodule=3  transfer=Blocking  dutycycle=TLow/THigh = 2  clkspeed=400  timeout=25  writecount=2  readcount=0  sdapin=C9  sclpin=A8  waitwritetime=0  forcestop=off  inputtypearray=[3 3 3 3]  outputtypearray=[1 3]  confstr="[\"C\",\"9\",\"A\",\"8\",\"1\",\"3\",\"4\",\"2\",\"I2C_DutyCycle_2\",\"0\",\"off\"]"  sampletime=-1  sampletimestr=0.008  blockid=ReadIMUAccelometerGyroscopeI2C3MPU9250InitWriteConfigurationI2CMasterReadWrite1
  INT_PIN_CFG1 : Constant  Value=hex2dec('37')  OutDataTypeStr=uint8  SampleTime=-1
  Terminator : Terminator
  wires:
  I2C Master Read/Write1/1 -> Terminator/1
  BYPASS_EN/1 -> I2C Master Read/Write1/3
  INT_PIN_CFG1/1 -> I2C Master Read/Write1/2
  SlvAddr/1 -> I2C Master Read/Write1/1

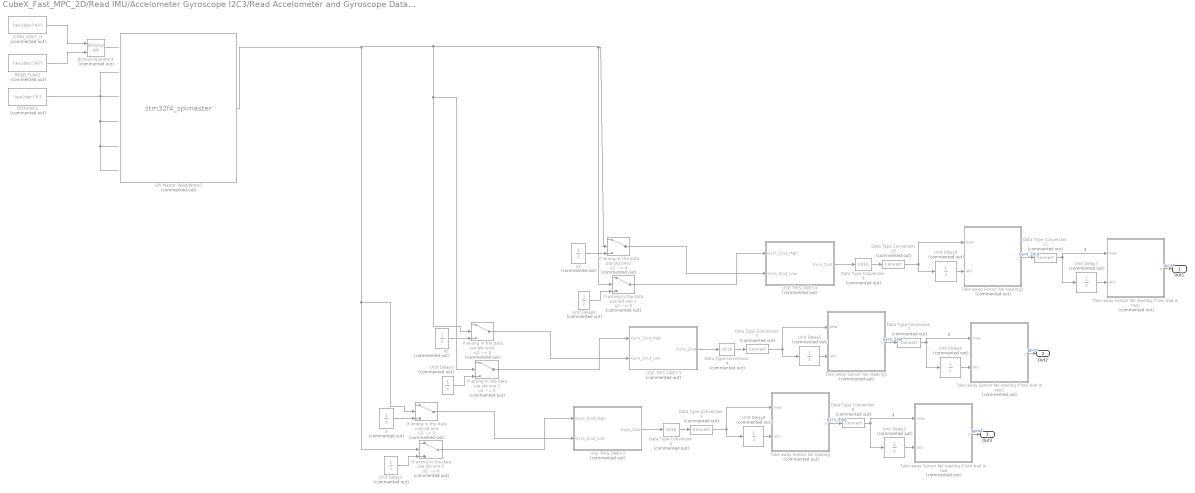
== system CubeX_Fast_MPC_2D/Read IMU/Accelometer Gyroscope I2C3/Read Accelometer and Gyroscope Data/Old gyro get data Used during SPI before ==
  " a" : UnitDelay  Commented=on  SampleTime=-1
  " a1" : UnitDelay  Commented=on  SampleTime=-1
  " a2" : UnitDelay  Commented=on  SampleTime=-1
  Bitwise Operator3 : simulink/Logic and Bit Operations/Bitwise Operator  Commented=on  logicop=OR  UseBitMask=off  NumInputPorts=2  BitMask=bin2dec('11011001')  BitMaskRealWorld=Stored Integer
  Data Type Conversion{3,5,7..8,10..11} (6 alike) : DataTypeConversion  Commented=on
  Data Type Conversion2 : DataTypeConversion  Commented=on  OutDataTypeStr=int16
  Data Type Conversion4 : DataTypeConversion  Commented=on  OutDataTypeStr=int16
  Data Type Conversion9 : DataTypeConversion  Commented=on  OutDataTypeStr=int16
  GYRO_XOUT_H : Constant  Commented=on  Value=hex2dec('43')  OutDataTypeStr=uint8
  If wrong in the data use old one : Switch  Commented=on  Criteria=u2 ~= 0
  If wrong in the data use old one 1 : Switch  Commented=on  Criteria=u2 ~= 0
  If wrong in the data use old one 2 : Switch  Commented=on  Criteria=u2 ~= 0
  If wrong in the data use old one 3 : Switch  Commented=on  Criteria=u2 ~= 0
  If wrong in the data use old one1 : Switch  Commented=on  Criteria=u2 ~= 0
  If wrong in the data use old one2 : Switch  Commented=on  Criteria=u2 ~= 0
  NOTHING1 : Constant  Commented=on  Value=hex2dec('0')  OutDataTypeStr=uint8
  READ_FLAG2 : Constant  Commented=on  Value=hex2dec('80')  OutDataTypeStr=uint8
  SPI Master Read/Write5 : S-Function  Commented=on  FunctionName=stm32f4_spimaster  Parameters=mode,configuration,module,datacount,inputtypearray,outputtypearray,confstr,sampletime,sampletimestr,blockid  SFunctionDeploymentMode=off  EnableBusSupport=off  mask(stm32f4_spimaster){configuration=Transaction, module=3, mode=Read/ Write, lastmodule=1, direction=Full-Duplex, dataformat=8bit/ FirstBit_MSB, prescaler=4, cpolcpha=CPOL_Low/ CPHA_1Edge, datacount='Could not find SPI Master Setup block for module 3', nssmode=Custom, nsspin=Not used, softnssport=E, softnsspin=0, sckpin=A5, misopin=A6, mosipin=A7, inputtypearray=[0], outputtypearray=[1 7], confstr=["SPI_Direction_2Lines_FullDuplex","8b","MSB","Low","1Edge","4","Soft","0","x","x","0","x","x","1","A","5","1","A","6","1","A","7","1","0","0","0","0","0","0","0","0","PP","0","UP"], sampletime=-1, sampletimestr=-1, blockid=AccelometerGyroscopeI2CReadAccelometerandGyroscopeDataOldgyrogetdataUsedduringSPIbeforeSPIMasterReadWrite5}
      mask prompts: module "SPI Module:"; lastmodule "Last module:"; dataformat "Data format:"; prescaler "Buad rate prescaler: Pclk/"; cpolcpha "Clock polarity (CPOL)/ Clock phase (CPHA):"; datacount "Data Read/Write count:"; nssmode "Slave/chip select (nSS, nCS) mode"; nsspin "Slave/chip select (nSS, nCS) pin"; softnssport "Slave/chip select port (nSS, nCS)"; softnsspin "Slave/chip select pin (nSS, nCS)"; sckpin "SCLK pin:"; misopin "MISO pin:"; mosipin "MOSI pin:"; inputtypearray "Input type array"; outputtypearray "Output type array"; confstr "Configuration string"; sampletime "Sample time (sec)"; sampletimestr "Compiled sample time (sec) in string"
      mask help:
      | Status:
      |  0 - Success.
      |  Otherwise - Fail.
      mask init:
      | stm32f4_spimaster_callback('init');
      mask Help: web(fullfile(waijungdocroot,'stm32f4_spimaster_readwrite.htm'), '-browser')
      mask TypeOptions configuration: Setup | Transaction
      mask Callback configuration: stm32f4_spimaster_callback('configuration');
      mask TypeOptions module: 1 | 2 | 3
      mask Callback module: stm32f4_spimaster_callback('module');
      mask TypeOptions mode: Read/ Write | Read | Write
      mask Callback mode: stm32f4_spimaster_callback('mode');
      mask TypeOptions direction: Full-Duplex | Half-Duplex_Tx | Half-Duplex_Rx
      mask Callback direction: stm32f4_spimaster_callback('direction');
      mask TypeOptions dataformat: 8bit/ FirstBit_MSB | 8bit/ FirstBit_LSB | 16bit/ FirstBit_MSB | 16bit/ FirstBit_LSB
      mask TypeOptions prescaler: 2 | 4 | 8 | 16 | 32 | 64 | 128 | 256
      mask TypeOptions cpolcpha: CPOL_Low/ CPHA_1Edge | CPOL_Low/ CPHA_2Edge | CPOL_High/ CPHA_1Edge | CPOL_High/ CPHA_2Edge
      mask Callback datacount: stm32f4_spimaster_callback('datacount');
      mask TypeOptions nssmode: Hardware | Software | Custom
      mask Callback nssmode: stm32f4_spimaster_callback('nssmode');
      mask TypeOptions nsspin: Not used | A4 | A15
      mask TypeOptions softnssport: A | B | C | D | E | F | G | H | I
      mask TypeOptions softnsspin: 0 | 1 | 2 | 3 | 4 | 5 | 6 | 7 | 8 | 9 | 10 | 11 | 12 | 13 | 14 | 15
      mask TypeOptions sckpin: Not used | A5 | B3
      mask TypeOptions misopin: Not used | A6 | B4
      mask TypeOptions mosipin: Not used | A7 | B5
      mask Callback confstr: stm32f4_spimaster_callback('confstr');
      mask Callback sampletime: stm32f4_spimaster_callback('sampletime');
      mask Callback sampletimestr: stm32f4_spimaster_callback('sampletimestr');
      mask Callback blockid: stm32f4_spimaster_callback('blockid');
      mask Display: text(0.5, 0.5, 'Module: SPI3 (Master)\nRead/ Write\nTs (sec): -1','ver','middle','hor','center');port_label('output', 1,'Status');
  Take away Sensor fail reading : MATLAB Function  Commented=on  TreatAsAtomicUnit=on
  Take away Sensor fail reading if two bad in raw : MATLAB Function  Commented=on  TreatAsAtomicUnit=on
  Take away Sensor fail reading if two bad in raw1 : MATLAB Function  Commented=on  TreatAsAtomicUnit=on
  Take away Sensor fail reading if two bad in raw2 : MATLAB Function  Commented=on  TreatAsAtomicUnit=on
  Take away Sensor fail reading1 : MATLAB Function  Commented=on  TreatAsAtomicUnit=on
  Take away Sensor fail reading2 : MATLAB Function  Commented=on  TreatAsAtomicUnit=on
  USE THIS ONE!!2 : Subsystem  Commented=on
  USE THIS ONE!!3 : Subsystem  Commented=on
  USE THIS ONE!!4 : Subsystem  Commented=on
  Unit Delay1 : UnitDelay  Commented=on  SampleTime=-1
  Unit Delay{2,4..5,7..9} (6 alike) : UnitDelay  Commented=on  InitialCondition=-40.45  SampleTime=-1
  Unit Delay3 : UnitDelay  Commented=on  SampleTime=-1
  Unit Delay6 : UnitDelay  Commented=on  SampleTime=-1
  Out1 : Outport
  Out2 : Outport  Port=2
  Out3 : Outport  Port=3
  wires:
  Data Type Conversion8/1 -> Unit Delay2/1, Take away Sensor fail reading if two bad in raw/1(new)  "3"
  Bitwise Operator3/1 -> ?
  USE THIS ONE!!2/1(Gyro_Zout) -> Data Type Conversion2/1
  GYRO_XOUT_H/1 -> Bitwise Operator3/1
  Unit Delay8/1 -> Take away Sensor fail reading/2(old)
  ? -> If wrong in the data use old one 2/1, Unit Delay1/1
  READ_FLAG2/1 -> Bitwise Operator3/2
  If wrong in the data use old one 2/1 -> USE THIS ONE!!2/1("Gyro_Zout_High ")
  If wrong in the data use old one/1 -> USE THIS ONE!!2/2(Gyro_Zout_Low)
  ? -> " a"/1, If wrong in the data use old one/1  "Gyro_zou_Lowt"
  " a"/1 -> If wrong in the data use old one/3
  Data Type Conversion2/1 -> Data Type Conversion3/1
  NOTHING1/1 -> ?
  Unit Delay1/1 -> If wrong in the data use old one 2/3
  Take away Sensor fail reading/1(y) -> Data Type Conversion8/1  "Gyro_Zout"
  Unit Delay2/1 -> Take away Sensor fail reading if two bad in raw/2(old)
  Unit Delay7/1 -> Take away Sensor fail reading if two bad in raw2/2(old)
  If wrong in the data use old one1/1 -> USE THIS ONE!!3/2(Gyro_Zout_Low)
  ? -> Unit Delay3/1, If wrong in the data use old one 1/1  "Gyro_zou_Lowt"
  " a2"/1 -> If wrong in the data use old one2/3
  Take away Sensor fail reading2/1(y) -> Data Type Conversion11/1  "Gyro_Zout"
  Data Type Conversion10/1 -> Take away Sensor fail reading2/1(new), Unit Delay9/1
  Data Type Conversion11/1 -> Unit Delay7/1, Take away Sensor fail reading if two bad in raw2/1(new)  "3"
  Unit Delay5/1 -> Take away Sensor fail reading1/2(old)
  SPI Master Read/Write5/1 -> If wrong in the data use old one2/2, If wrong in the data use old one 3/2, If wrong in the data use old one 1/2, If wrong in the data use old one1/2, If wrong in the data use old one 2/2, If wrong in the data use old one/2
  ? -> " a2"/1, If wrong in the data use old one2/1  "Gyro_zou_Lowt"
  ? -> " a1"/1, If wrong in the data use old one1/1  "Gyro_zou_Lowt"
  Data Type Conversion7/1 -> Unit Delay4/1, Take away Sensor fail reading if two bad in raw1/1(new)  "3"
  Data Type Conversion3/1 -> Take away Sensor fail reading/1(new), Unit Delay8/1
  Data Type Conversion4/1 -> Data Type Conversion5/1
  Data Type Conversion9/1 -> Data Type Conversion10/1
  USE THIS ONE!!3/1(Gyro_Zout) -> Data Type Conversion4/1
  " a1"/1 -> If wrong in the data use old one1/3
  Unit Delay6/1 -> If wrong in the data use old one 3/3
  USE THIS ONE!!4/1(Gyro_Zout) -> Data Type Conversion9/1
  If wrong in the data use old one 1/1 -> USE THIS ONE!!3/1("Gyro_Zout_High ")
  If wrong in the data use old one2/1 -> USE THIS ONE!!4/2(Gyro_Zout_Low)
  Unit Delay3/1 -> If wrong in the data use old one 1/3
  Data Type Conversion5/1 -> Take away Sensor fail reading1/1(new), Unit Delay5/1
  ? -> If wrong in the data use old one 3/1, Unit Delay6/1  "Gyro_zou_Lowt"
  If wrong in the data use old one 3/1 -> USE THIS ONE!!4/1("Gyro_Zout_High ")
  Unit Delay9/1 -> Take away Sensor fail reading2/2(old)
  Unit Delay4/1 -> Take away Sensor fail reading if two bad in raw1/2(old)
  Take away Sensor fail reading1/1(y) -> Data Type Conversion7/1  "Gyro_Zout"
  Take away Sensor fail reading if two bad in raw2/1(y) -> Out1/1  "gyroX"
  Take away Sensor fail reading if two bad in raw/1(y) -> Out3/1  "gyroZ"
  Take away Sensor fail reading if two bad in raw1/1(y) -> Out2/1  "gyroY"

== system CubeX_Fast_MPC_2D/Read IMU/Accelometer Gyroscope I2C3/Read Accelometer and Gyroscope Data/Turn the MSB and LSB into a signed 16-bit integer AccX ==
  note: Bitshift up the MSB bits and bitwise OR the LSB
      | into a int16
  MSB : Inport
  LSB : Inport  Port=2
  Bitwise Operator2 : simulink/Logic and Bit Operations/Bitwise Operator  logicop=OR  UseBitMask=off  NumInputPorts=2  BitMask=bin2dec('11011001')  BitMaskRealWorld=Stored Integer
  Data Type Conversion6 : DataTypeConversion  OutDataTypeStr=uint16
  Data Type Conversion7 : DataTypeConversion  OutDataTypeStr=uint16
  Shift Arithmetic2 : ArithShift  BitShiftNumber=-8
  out16b : Outport
  wires:
  LSB/1 -> Data Type Conversion6/1
  Bitwise Operator2/1 -> out16b/1
  MSB/1 -> Data Type Conversion7/1
  Data Type Conversion7/1 -> Shift Arithmetic2/1
  Data Type Conversion6/1 -> Bitwise Operator2/2
  Shift Arithmetic2/1 -> Bitwise Operator2/1

== system CubeX_Fast_MPC_2D/Read IMU/Accelometer Gyroscope I2C3/Read Accelometer and Gyroscope Data/Turn the MSB and LSB into a signed 16-bit integer AccY ==
  note: Bitshift up the MSB bits and bitwise OR the LSB
      | into a int16
  MSB : Inport
  LSB : Inport  Port=2
  Bitwise Operator2 : simulink/Logic and Bit Operations/Bitwise Operator  logicop=OR  UseBitMask=off  NumInputPorts=2  BitMask=bin2dec('11011001')  BitMaskRealWorld=Stored Integer
  Data Type Conversion6 : DataTypeConversion  OutDataTypeStr=uint16
  Data Type Conversion7 : DataTypeConversion  OutDataTypeStr=uint16
  Shift Arithmetic2 : ArithShift  BitShiftNumber=-8
  out16b : Outport
  wires:
  LSB/1 -> Data Type Conversion6/1
  Bitwise Operator2/1 -> out16b/1
  MSB/1 -> Data Type Conversion7/1
  Data Type Conversion7/1 -> Shift Arithmetic2/1
  Data Type Conversion6/1 -> Bitwise Operator2/2
  Shift Arithmetic2/1 -> Bitwise Operator2/1

== system CubeX_Fast_MPC_2D/Read IMU/Accelometer Gyroscope I2C3/Read Accelometer and Gyroscope Data/Turn the MSB and LSB into a signed 16-bit integer AccZ ==
  note: Bitshift up the MSB bits and bitwise OR the LSB
      | into a int16
  MSB : Inport
  LSB : Inport  Port=2
  Bitwise Operator2 : simulink/Logic and Bit Operations/Bitwise Operator  logicop=OR  UseBitMask=off  NumInputPorts=2  BitMask=bin2dec('11011001')  BitMaskRealWorld=Stored Integer
  Data Type Conversion6 : DataTypeConversion  OutDataTypeStr=uint16
  Data Type Conversion7 : DataTypeConversion  OutDataTypeStr=uint16
  Shift Arithmetic2 : ArithShift  BitShiftNumber=-8
  out16b : Outport
  wires:
  LSB/1 -> Data Type Conversion6/1
  Bitwise Operator2/1 -> out16b/1
  MSB/1 -> Data Type Conversion7/1
  Data Type Conversion7/1 -> Shift Arithmetic2/1
  Data Type Conversion6/1 -> Bitwise Operator2/2
  Shift Arithmetic2/1 -> Bitwise Operator2/1

== system CubeX_Fast_MPC_2D/Read IMU/Accelometer Gyroscope I2C3/Read Accelometer and Gyroscope Data/Turn the MSB and LSB into a signed 16-bit integer GyroX ==
  note: Bitshift up the MSB bits and bitwise OR the LSB
      | into a int16
  MSB : Inport
  LSB : Inport  Port=2
  Bitwise Operator2 : simulink/Logic and Bit Operations/Bitwise Operator  logicop=OR  UseBitMask=off  NumInputPorts=2  BitMask=bin2dec('11011001')  BitMaskRealWorld=Stored Integer
  Data Type Conversion6 : DataTypeConversion  OutDataTypeStr=uint16
  Data Type Conversion7 : DataTypeConversion  OutDataTypeStr=uint16
  Shift Arithmetic2 : ArithShift  BitShiftNumber=-8
  out16b : Outport
  wires:
  LSB/1 -> Data Type Conversion6/1
  Bitwise Operator2/1 -> out16b/1
  MSB/1 -> Data Type Conversion7/1
  Data Type Conversion7/1 -> Shift Arithmetic2/1
  Data Type Conversion6/1 -> Bitwise Operator2/2
  Shift Arithmetic2/1 -> Bitwise Operator2/1

== system CubeX_Fast_MPC_2D/Read IMU/Accelometer Gyroscope I2C3/Read Accelometer and Gyroscope Data/Turn the MSB and LSB into a signed 16-bit integer GyroY ==
  note: Bitshift up the MSB bits and bitwise OR the LSB
      | into a int16
  MSB : Inport
  LSB : Inport  Port=2
  Bitwise Operator2 : simulink/Logic and Bit Operations/Bitwise Operator  logicop=OR  UseBitMask=off  NumInputPorts=2  BitMask=bin2dec('11011001')  BitMaskRealWorld=Stored Integer
  Data Type Conversion6 : DataTypeConversion  OutDataTypeStr=uint16
  Data Type Conversion7 : DataTypeConversion  OutDataTypeStr=uint16
  Shift Arithmetic2 : ArithShift  BitShiftNumber=-8
  out16b : Outport
  wires:
  LSB/1 -> Data Type Conversion6/1
  Bitwise Operator2/1 -> out16b/1
  MSB/1 -> Data Type Conversion7/1
  Data Type Conversion7/1 -> Shift Arithmetic2/1
  Data Type Conversion6/1 -> Bitwise Operator2/2
  Shift Arithmetic2/1 -> Bitwise Operator2/1

== system CubeX_Fast_MPC_2D/Read IMU/Accelometer Gyroscope I2C3/Read Accelometer and Gyroscope Data/Turn the MSB and LSB into a signed 16-bit integer GyroZ ==
  note: Bitshift up the MSB bits and bitwise OR the LSB
      | into a int16
  MSB : Inport
  LSB : Inport  Port=2
  Bitwise Operator2 : simulink/Logic and Bit Operations/Bitwise Operator  logicop=OR  UseBitMask=off  NumInputPorts=2  BitMask=bin2dec('11011001')  BitMaskRealWorld=Stored Integer
  Data Type Conversion6 : DataTypeConversion  OutDataTypeStr=uint16
  Data Type Conversion7 : DataTypeConversion  OutDataTypeStr=uint16
  Shift Arithmetic2 : ArithShift  BitShiftNumber=-8
  out16b : Outport
  wires:
  LSB/1 -> Data Type Conversion6/1
  Bitwise Operator2/1 -> out16b/1
  MSB/1 -> Data Type Conversion7/1
  Data Type Conversion7/1 -> Shift Arithmetic2/1
  Data Type Conversion6/1 -> Bitwise Operator2/2
  Shift Arithmetic2/1 -> Bitwise Operator2/1
